simulink model "Question2"  (R2017a)
settings: Solver=VariableStepAuto  StartTime=0.0  StopTime=10.0  RelTol=1e-3
settings Model: Creator=ALI  LastModifiedBy=ALI

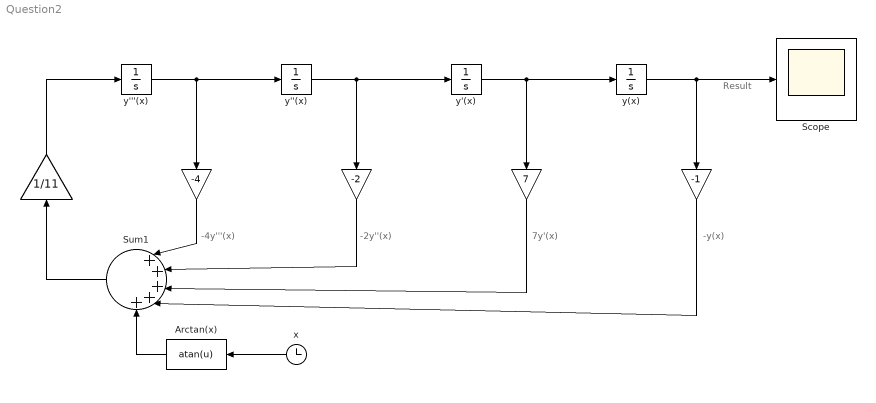
== system Question2 ==
  note: Result
  note: -y(x)
  note: 7y'(x)
  note: -2y''(x)
  note: -4y'''(x)
  " " : Gain  Gain=1/11
  "  " : Gain  Gain=-4
  "   " : Gain  Gain=-2
  "    " : Gain  Gain=7
  "     " : Gain  Gain=-1
  Arctan(x) : Fcn  Expr=atan(u)
  Scope : Scope
  Sum1 : Sum  Inputs=|+++++
  x : Clock
  y'''(x) : Integrator
  y''(x) : Integrator
  y'(x) : Integrator
  y(x) : Integrator
  wires:
  x/1 -> Arctan(x)/1
  y'''(x)/1 -> "  "/1, y''(x)/1
  y''(x)/1 -> "   "/1, y'(x)/1
  y'(x)/1 -> "    "/1, y(x)/1
  y(x)/1 -> Scope/1, "     "/1
  Arctan(x)/1 -> Sum1/5
  "     "/1 -> Sum1/4
  " "/1 -> y'''(x)/1
  "    "/1 -> Sum1/3
  "   "/1 -> Sum1/2
  "  "/1 -> Sum1/1
  Sum1/1 -> " "/1
